simulink model "bpsk_rx7"  (R2021b)
settings: Solver=FixedStepDiscrete  StartTime=0.0  StopTime=2000  RelTol=1e-3
libraries: dsp_blocks x10
settings Model: Creator=aidynardabek  LastModifiedBy=aidynardabek

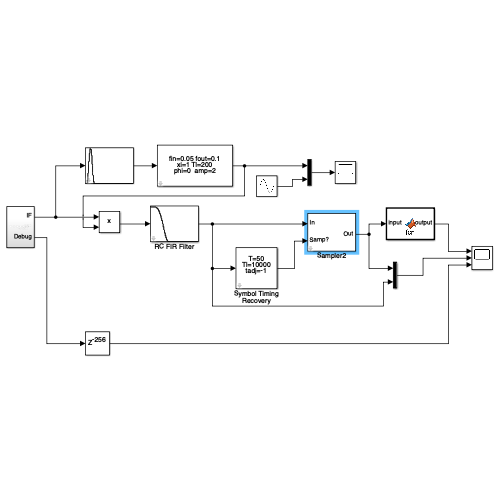
[thumbnail: Simulink's stored preview of the top-level diagram]
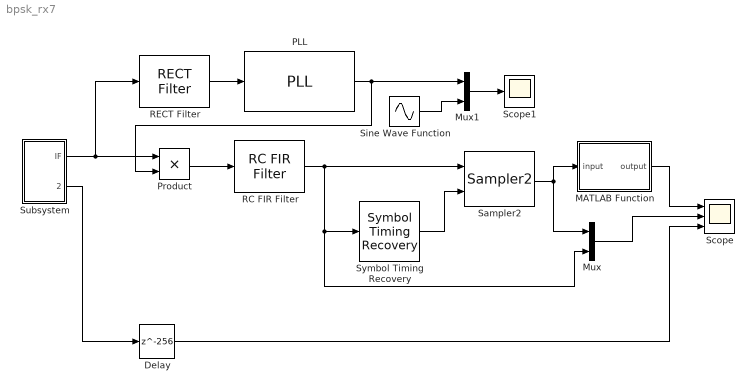
== system bpsk_rx7 ==
  Delay : Delay  DelayLength=256  InitialCondition=0
  MATLAB Function : MATLAB Function  TreatAsAtomicUnit=on
  Mux : Mux  Inputs=2
  Mux1 : Mux  Inputs=2
  PLL : dsp_blocks/Timing /PLL  freq=0.05  freq_out=0.1  phi=0  amp=2  xi=1  K=2  T=200
  Product : Product
  RC FIR Filter : dsp_blocks/Filters/RC FIR Filter  period=50  beta=0.5  root=on  filt_len=512  win_type=on
  RECT Filter : dsp_blocks/Filters/RECT Filter  f0=0.03  f1=0.07  filt_len=80
  Sampler2 : dsp_blocks/Conversions/Sampler2
  Scope : Scope  NumInputPorts=3
  Scope1 : Scope
  Sine Wave Function : Sin  Amplitude=2  Frequency=2*pi*0.1  SampleTime=0
  Subsystem : Subsystem
  Symbol Timing Recovery : dsp_blocks/Timing /Symbol Timing Recovery  T=50  Tl=10000  tadj=-1
  wires:
  Subsystem/1(IF) -> RECT Filter/1, Product/1
  Subsystem/2(Debug) -> Delay/1
  Product/1 -> RC FIR Filter/1
  RC FIR Filter/1 -> Sampler2/1, Symbol Timing Recovery/1, Mux/2
  Sampler2/1 -> MATLAB Function/1(input), Mux/1
  MATLAB Function/1(output) -> Scope/1
  Delay/1 -> Scope/3
  Mux/1 -> Scope/2
  RECT Filter/1 -> PLL/1
  Sine Wave Function/1 -> Mux1/2
  PLL/1 -> Product/2, Mux1/1
  Mux1/1 -> Scope1/1
  Symbol Timing Recovery/1 -> Sampler2/2

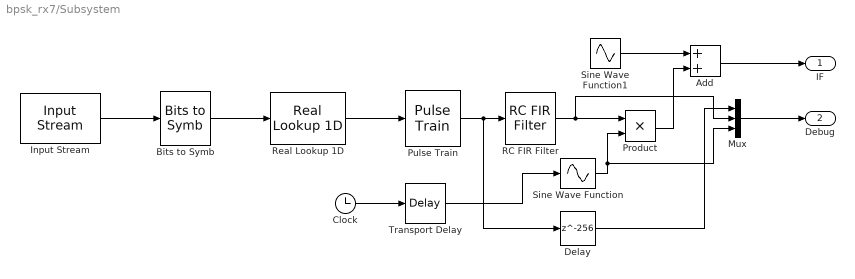
== system bpsk_rx7/Subsystem ==
  Add : Sum
  Bits to Symb : dsp_blocks/Conversions/Bits to Symb
  Clock : Clock
  Delay : Delay  DelayLength=256
  Input Stream : dsp_blocks/Sources//Sinks/Input Stream  period=50  width=1  fname=rand.mat
  Mux : Mux  Inputs=3
  Product : Product
  Pulse Train : dsp_blocks/Conversions/Pulse Train  period=50
  RC FIR Filter : dsp_blocks/Filters/RC FIR Filter  period=50  beta=0.5  root=on  filt_len=512  win_type=on
  Real Lookup 1D : dsp_blocks/Conversions/Real Lookup 1D  table=[-1 1]
  Sine Wave Function : Sin  TimeSource=Use external signal  Frequency=2*pi*0.1  SampleTime=0
  Sine Wave Function1 : Sin  Amplitude=0.05  Frequency=2*pi*0.05  SampleTime=0
  Transport Delay : TransportDelay
  IF : Outport
  Debug : Outport  Port=2
  wires:
  Delay/1 -> Mux/1
  Mux/1 -> Debug/1
  Bits to Symb/1 -> Real Lookup 1D/1
  RC FIR Filter/1 -> Mux/2, Product/1
  Input Stream/1 -> Bits to Symb/1
  Real Lookup 1D/1 -> Pulse Train/1
  Sine Wave Function/1 -> Mux/3, Product/2
  Pulse Train/1 -> Delay/1, RC FIR Filter/1
  Clock/1 -> Transport Delay/1
  Transport Delay/1 -> Sine Wave Function/1
  Sine Wave Function1/1 -> Add/1
  Product/1 -> Add/2
  Add/1 -> IF/1

== matlab function bpsk_rx7/MATLAB Function ==
  data: input input; output output
function output = fcn(input)

if (input > 0)
    output = 1;
else
    output = 0;
end
